simulink model "Thomas"  (R2014b)
settings: Solver=ode45  StartTime=0.0  StopTime=10.0  RelTol=1e-3
values from neighbouring files (symbols this model uses):
  b = 0.7    [Run_Aizawa.m]    (also in Run_Arneodo.m = 3.5; Run_Chen.m = 3; Run_Chua.m = 28; Run_Duffing.m = 100)
undefined symbols (not defined in the file or in its folder): param
settings Model: Creator=Arek  LastModifiedBy=Arek

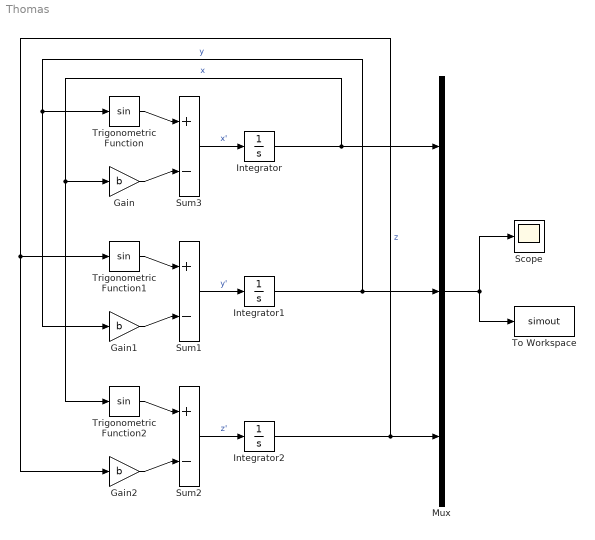
== system Thomas ==
  Gain : Gain  Gain=b
  Gain1 : Gain  Gain=b
  Gain2 : Gain  Gain=b
  Integrator : Integrator  InitialCondition=param.ic(1)
  Integrator1 : Integrator  InitialCondition=param.ic(2)
  Integrator2 : Integrator  InitialCondition=param.ic(3)
  Mux : Mux  Inputs=3
  Scope : Scope
      settings: ShowLegends=on
  Sum1 : Sum  Inputs=+|-
  Sum2 : Sum  Inputs=+|-
  Sum3 : Sum  Inputs=+|-
  To Workspace : ToWorkspace  VariableName=simout  SaveFormat=Timeseries  SampleTime=-1
  Trigonometric Function : Trigonometry
  Trigonometric Function1 : Trigonometry
  Trigonometric Function2 : Trigonometry
  wires:
  Integrator/1 -> Trigonometric Function2/1, Gain/1, Mux/1  "x"
  Sum1/1 -> Integrator1/1  "y'"
  Integrator1/1 -> Mux/2, Trigonometric Function/1, Gain1/1  "y"
  Sum2/1 -> Integrator2/1  "z'"
  Integrator2/1 -> Mux/3, Gain2/1, Trigonometric Function1/1  "z"
  Mux/1 -> Scope/1, To Workspace/1
  Sum3/1 -> Integrator/1  "x'"
  Gain/1 -> Sum3/2
  Trigonometric Function/1 -> Sum3/1
  Gain1/1 -> Sum1/2
  Trigonometric Function1/1 -> Sum1/1
  Gain2/1 -> Sum2/2
  Trigonometric Function2/1 -> Sum2/1
